simulink model "s0314"  (Simulink 6.0)
settings: Solver=ode3  SolverMode=SingleTasking  StartTime=0.0  StopTime=900  FixedStep=1  MaxStep=1  RelTol=1e-3  AbsTol=1e-6
values from neighbouring files (symbols this model uses):
  Kps = 1    [m0305.m]    (also in m0306.m; m0311.m; m0313.m; m0314.m = 0.143)
  nen = Gs.den{1}    [m0251.m]    (also in m0252.m; m0256.m; m0258.m; m0304.m = G.den{1})
  T1 = 3*T1    (= 0.3)    [m0203.m]    (also in m0204.m = 0.1; m0205.m = 0.1; m0207.m = 0.1; m0221d.m = 1/a0)
  T1m = b*V*R/2    (= 0.5)    [m0314.m]
  Tt = .4    (= 0.4)    [m0108d.m]    (also in m0259.m = 1; m0314.m = 2.13; m0322.m = 0.8; m0326.m = 4)
  Ttu = .13    (= 0.13)    [m0314.m]
  ydach = 1    [m0305.m]    (also in m0306.m; m0311.m; m0312b.m; m0313.m)
  zae = Gs.num{1}    [m0251.m]    (also in m0252.m; m0256.m; m0258.m; m0304.m = G.num{1})
settings Model: LastModifiedBy=Froriep
settings DataIOCC: LimitDataPoints=off  SaveOutput=off  SaveTime=off
settings OptimizationCC: BooleanDataType=off
settings DebuggingCC: SolverPrmCheckMsg=none
settings HardwareCC: TargetUnknown=on
settings GRTTargetCC: ModelReferenceCompliant=off  MatFileLogging=off

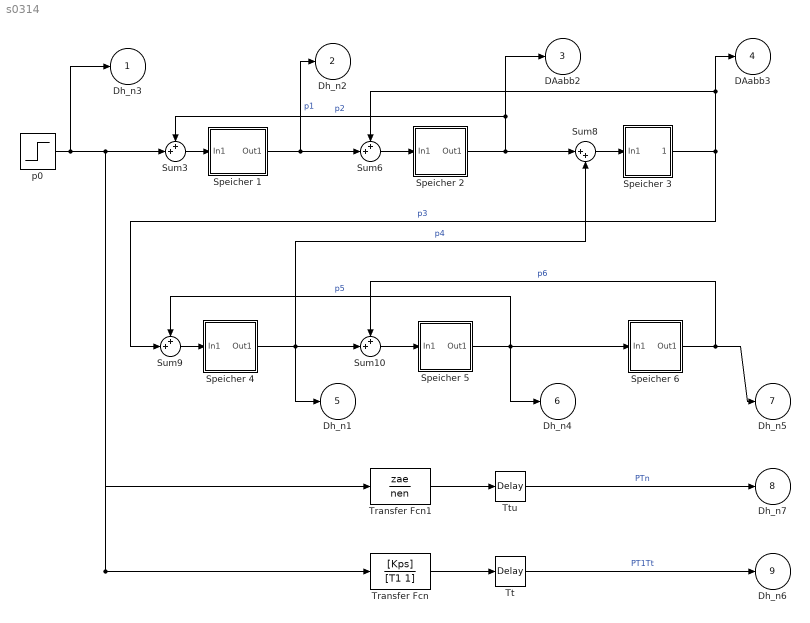
== system s0314 ==
  Speicher 1 : Subsystem
  Speicher 2 : Subsystem
  Speicher 3 : Subsystem
  Speicher 4 : Subsystem
  Speicher 5 : Subsystem
  Speicher 6 : Subsystem
  Sum{3,6,9..10} (4 alike) : Sum  Inputs=++|
  Sum8 : Sum  Inputs=|++
  Transfer Fcn : TransferFcn  Numerator=[Kps]  Denominator=[T1 1]
  Transfer Fcn1 : TransferFcn  Numerator=zae  Denominator=nen
  Tt : TransportDelay  DelayTime=Tt
  Ttu : TransportDelay  DelayTime=Ttu
  p0 : Step  Time=0  After=ydach  SampleTime=0
  Dh_n3 : Outport
  Dh_n2 : Outport  Port=2
  DAabb2 : Outport  Port=3
  DAabb3 : Outport  Port=4
  Dh_n1 : Outport  Port=5
  Dh_n4 : Outport  Port=6
  Dh_n5 : Outport  Port=7
  Dh_n7 : Outport  Port=8
  Dh_n6 : Outport  Port=9
  wires:
  Sum3/1 -> Speicher 1/1(In1)
  p0/1 -> Dh_n3/1, Sum3/2, Transfer Fcn/1, Transfer Fcn1/1
  Sum6/1 -> Speicher 2/1(In1)
  Transfer Fcn/1 -> Tt/1
  Tt/1 -> Dh_n6/1  "PT1Tt"
  Sum8/1 -> Speicher 3/1(In1)
  Sum9/1 -> Speicher 4/1(In1)
  Sum10/1 -> Speicher 5/1(In1)
  Speicher 1/1(Out1) -> Sum6/2, Dh_n2/1  "p1"
  Speicher 2/1(Out1) -> DAabb2/1, Sum3/1, Sum8/1  "p2"
  Speicher 3/1(Out1) -> DAabb3/1, Sum6/1, Sum9/2  "p3"
  Speicher 4/1(Out1) -> Sum10/2, Sum8/2, Dh_n1/1  "p4"
  Speicher 5/1(Out1) -> Speicher 6/1(In1), Dh_n4/1, Sum9/1  "p5"
  Speicher 6/1(Out1) -> Dh_n5/1, Sum10/1  "p6"
  Transfer Fcn1/1 -> Ttu/1
  Ttu/1 -> Dh_n7/1  "PTn"

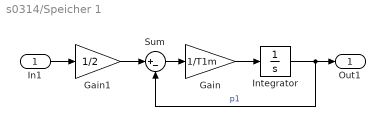
== system s0314/Speicher 1 ==
  In1 : Inport  Port=1  LatchInput=off
  Gain : Gain  Gain=1/T1m
  Gain1 : Gain  Gain=1/2
  Integrator : Integrator
  Sum : Sum  Inputs=|+-
  Out1 : Outport
  wires:
  Gain1/1 -> Sum/1
  Integrator/1 -> Sum/2, Out1/1  "p1"
  Sum/1 -> Gain/1
  Gain/1 -> Integrator/1
  In1/1 -> Gain1/1

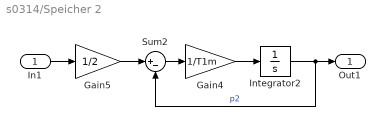
== system s0314/Speicher 2 ==
  In1 : Inport  Port=1  LatchInput=off
  Gain4 : Gain  Gain=1/T1m
  Gain5 : Gain  Gain=1/2
  Integrator2 : Integrator
  Sum2 : Sum  Inputs=|+-
  Out1 : Outport
  wires:
  Gain4/1 -> Integrator2/1
  Sum2/1 -> Gain4/1
  Integrator2/1 -> Sum2/2, Out1/1  "p2"
  Gain5/1 -> Sum2/1
  In1/1 -> Gain5/1

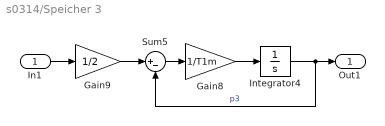
== system s0314/Speicher 3 ==
  In1 : Inport  Port=1  LatchInput=off
  Gain8 : Gain  Gain=1/T1m
  Gain9 : Gain  Gain=1/2
  Integrator4 : Integrator
  Sum5 : Sum  Inputs=|+-
  Out1 : Outport
  wires:
  Gain8/1 -> Integrator4/1
  Sum5/1 -> Gain8/1
  Integrator4/1 -> Sum5/2, Out1/1  "p3"
  Gain9/1 -> Sum5/1
  In1/1 -> Gain9/1

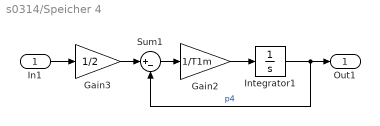
== system s0314/Speicher 4 ==
  In1 : Inport  Port=1  LatchInput=off
  Gain2 : Gain  Gain=1/T1m
  Gain3 : Gain  Gain=1/2
  Integrator1 : Integrator
  Sum1 : Sum  Inputs=|+-
  Out1 : Outport
  wires:
  Gain2/1 -> Integrator1/1
  Sum1/1 -> Gain2/1
  Integrator1/1 -> Sum1/2, Out1/1  "p4"
  Gain3/1 -> Sum1/1
  In1/1 -> Gain3/1

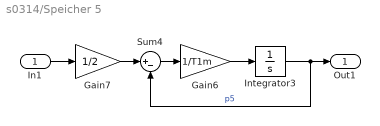
== system s0314/Speicher 5 ==
  In1 : Inport  Port=1  LatchInput=off
  Gain6 : Gain  Gain=1/T1m
  Gain7 : Gain  Gain=1/2
  Integrator3 : Integrator
  Sum4 : Sum  Inputs=|+-
  Out1 : Outport
  wires:
  Gain6/1 -> Integrator3/1
  Sum4/1 -> Gain6/1
  Integrator3/1 -> Sum4/2, Out1/1  "p5"
  Gain7/1 -> Sum4/1
  In1/1 -> Gain7/1

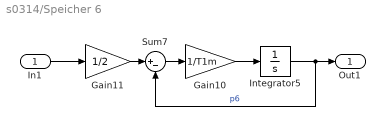
== system s0314/Speicher 6 ==
  In1 : Inport  Port=1  LatchInput=off
  Gain10 : Gain  Gain=1/T1m
  Gain11 : Gain  Gain=1/2
  Integrator5 : Integrator
  Sum7 : Sum  Inputs=|+-
  Out1 : Outport
  wires:
  Gain10/1 -> Integrator5/1
  Sum7/1 -> Gain10/1
  Integrator5/1 -> Sum7/2, Out1/1  "p6"
  Gain11/1 -> Sum7/1
  In1/1 -> Gain11/1
